simulink model "pokus05_serial_port"  (R2023a)
settings: Solver=VariableStepDiscrete  StartTime=0.0  StopTime=inf  RelTol=1e-3
undefined symbols (not defined in the file): UartDataRx, UartDataRx_Active
libraries: Miscellaneous x18, Memory_Blocks_Lib x7, Counters_Lib x4, Bit_Multiplexers_Lib x3, Decoders_Lib x2, Garbage x1, simulink_extras x1
settings Model: PacingRate=100  Creator=Jozko Mrkvicka  LastModifiedBy=Jozko Mrkvicka

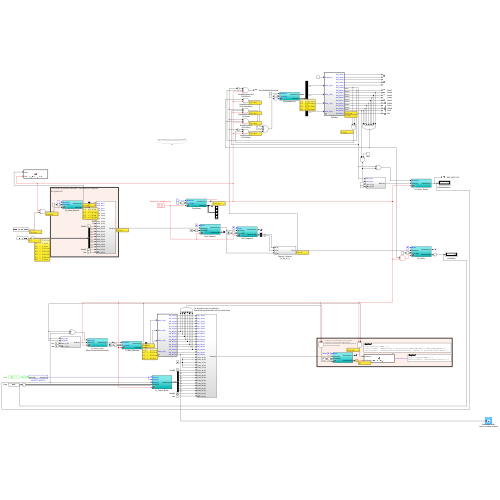
[thumbnail: Simulink's stored preview of the top-level diagram]
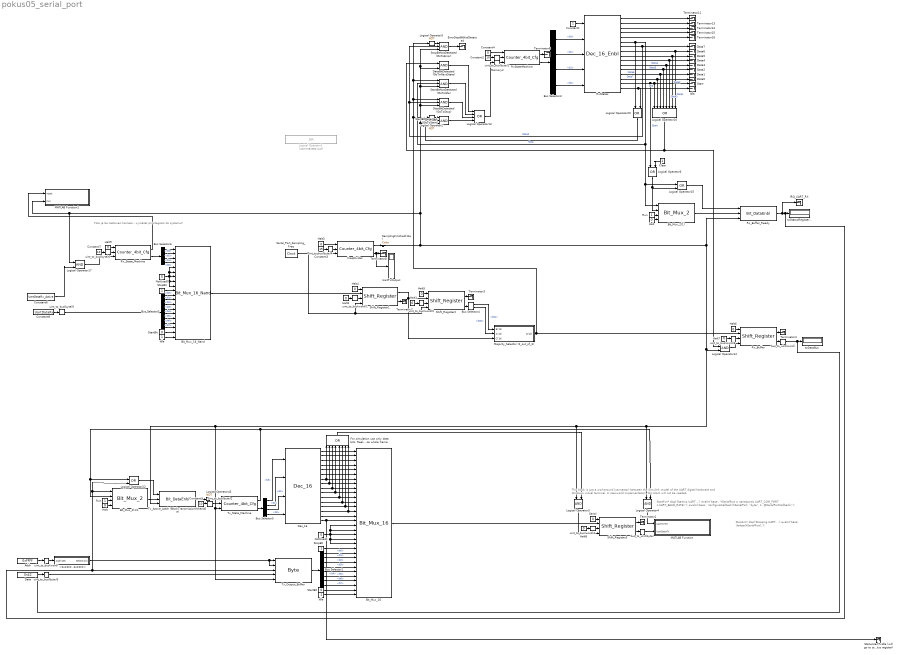
== system pokus05_serial_port ==
  note: Toto je len testovaci harness - vymazat pri integracii
      | do systemu!!
  note: StartFcn*
      | disp('Starting UART...')
      | evalin('base', 'hSerialPort = serialport(c.UART_COM_PORT, c.UART_BAUD_RATE);');
      | evalin('base', 'configureCallback(hSerialPort, "byte", 1, @SerialPortCallback);');
  note: StopFcn*
      | disp('Stopping UART...')
      | evalin('base', 'delete(hSerialPort);');
  note: This block is just a workaround (connector) between
      |                      the Simulink model of the UART digital hardware
      |                      and Windows virtual terminal. In real-world implementation,
      |                      this block will not be needed.
  "  Halt" : Constant  Value=0  OutDataTypeStr=boolean
  "  Idle" : Constant  OutDataTypeStr=boolean
   Halt{,3..6,9} (6 alike) : Constant  Value=0  OutDataTypeStr=boolean
   Halt{1..2,7..8} (4 alike) : Constant  Value=0  OutDataTypeStr=uint16
  " Idle" : Constant  OutDataTypeStr=boolean
  " Run" : Constant  OutDataTypeStr=boolean
  " StartBit" : Constant  Value=0  OutDataTypeStr=boolean
  " StopBit" : Constant  OutDataTypeStr=boolean
  <0xFFFF..0xFFFF> : Subsystem
  Addr : Constant  Value=0xFFFF  OutDataTypeStr=uint16
  Bit_Mux_16 : Bit_Multiplexers_Lib/Bit_Mux_16  SystemSampleTime=-1  VariantActivationTime=update diagram  Latency=0  AutoFrameSizeCalculation=off
  Bit_Mux_16_Nand : Garbage/Bit_Mux_16_Nand  SystemSampleTime=-1  VariantActivationTime=update diagram  Latency=0  AutoFrameSizeCalculation=off
  Bit_Mux_2(1) : Bit_Multiplexers_Lib/Bit_Mux_2  SystemSampleTime=-1  VariantActivationTime=update diagram  Latency=0  AutoFrameSizeCalculation=off
  Bit_Mux_2(1)1 : Bit_Multiplexers_Lib/Bit_Mux_2  SystemSampleTime=-1  VariantActivationTime=update diagram  Latency=0  AutoFrameSizeCalculation=off
  Bus Selector1 : BusSelector  OutputSignals=b0,b1,b2,b3,b4,b5,b6,b7
  Bus Selector2 : BusSelector  OutputSignals=b0,b1,b2,b3,b4,b5,b6,b7
  Bus Selector3 : BusSelector  OutputSignals=b3,b2,b1,b0
  Bus Selector4 : BusSelector  OutputSignals=b01,b00
  Bus Selector5 : BusSelector  OutputSignals=b3,b2,b1,b0
  Bus Selector6 : BusSelector  OutputSignals=b3,b2,b1,b0
  Clear : Constant  OutDataTypeStr=boolean
  Constant1 : Constant  OutDataTypeStr=boolean
  Constant2 : Constant  Value=10  OutDataTypeStr=uint8
  Constant3 : Constant  Value=15  OutDataTypeStr=uint8
  Constant4 : Constant  Value=0  OutDataTypeStr=boolean
  Constant5 : Constant  Value=10  OutDataTypeStr=uint8
  Constant6 : Constant  Value=UartDataRx_Active  OutDataTypeStr=boolean
  Constant7 : Constant  Value=10  OutDataTypeStr=uint8
  Constant8 : Constant  Value=UartDataRx  OutDataTypeStr=uint8
  Data : Constant  Value=0x42  OutDataTypeStr=uint8
  Data{0..7} (8 alike) : Terminator
  DataBitDetected (GoToNextState) : Logic  IconShape=distinctive  AllPortsSameDT=off  OutDataTypeStr=boolean
  Dec_16 : Decoders_Lib/Dec_16  SystemSampleTime=-1  VariantActivationTime=update diagram  Latency=0  AutoFrameSizeCalculation=off
  ErrorStopBitNotDetected : Terminator
  For simulation use only data bits. Real-world implementation will use whole frame. : Logic  Operator=OR  Inputs=8  IconShape=distinctive  AllPortsSameDT=off  OutDataTypeStr=boolean
  FreqDivider : Counters_Lib/Counter_4bit_Cfg  SystemSampleTime=-1  VariantActivationTime=update diagram  Latency=0  AutoFrameSizeCalculation=off
  IRQ_UART_RX : Terminator
  Idle : Terminator
  Logical Operator1 : Logic  Commented=on  Operator=OR  Inputs=16  IconShape=distinctive  OutDataTypeStr=boolean
  Logical Operator10 : Logic  Operator=OR  Inputs=8  IconShape=distinctive  AllPortsSameDT=off  OutDataTypeStr=boolean
  Logical Operator{3..4,12,17} (4 alike) : Logic  IconShape=distinctive  AllPortsSameDT=off  OutDataTypeStr=boolean
  Logical Operator13 : Logic  Operator=OR  Inputs=4  IconShape=distinctive  AllPortsSameDT=off  OutDataTypeStr=boolean
  Logical Operator{6,15,20,22} (4 alike) : Logic  Operator=OR  IconShape=distinctive  AllPortsSameDT=off  OutDataTypeStr=boolean
  Logical Operator2 : Logic  Operator=NOT  IconShape=distinctive  AllPortsSameDT=off  OutDataTypeStr=boolean
  Logical Operator43 : Logic  Operator=NOT  IconShape=distinctive  AllPortsSameDT=off  OutDataTypeStr=boolean
  Logical Operator5 : Logic  Operator=NOT  IconShape=distinctive  AllPortsSameDT=off  OutDataTypeStr=boolean
  MATLAB Function : MATLAB Function  StartFcn=|  StopFcn=|  TreatAsAtomicUnit=on  SystemSampleTime=1
      StartFcn=|
      | disp('Starting UART...')
      | evalin('base', 'hSerialPort = serialport(c.UART_COM_PORT, c.UART_BAUD_RATE);');
      | evalin('base', 'configureCallback(hSerialPort, "byte", 1, @SerialPortCallback);');
      StopFcn=|
      | disp('Stopping UART...')
      | evalin('base', 'delete(hSerialPort);');
  MATLAB Function1 : MATLAB Function  TreatAsAtomicUnit=on
  Majority_Selector (2_out_of_3) : Subsystem
  Memory2 : Memory
  NotUsed0 : Constant  Value=0  OutDataTypeStr=boolean
  NotUsed1 : Constant  Value=0  OutDataTypeStr=boolean
  Run : Constant  OutDataTypeStr=boolean
  RxStateMachine : Counters_Lib/Counter_4bit_Cfg  SystemSampleTime=-1  VariantActivationTime=update diagram  Latency=0  AutoFrameSizeCalculation=off
  RxStates : Decoders_Lib/Dec_16_Enbl  SystemSampleTime=-1  VariantActivationTime=update diagram  Latency=0  AutoFrameSizeCalculation=off
  Rx_Buffer : Memory_Blocks_Lib/Shift_Register  SystemSampleTime=-1  VariantActivationTime=update diagram  Latency=0  AutoFrameSizeCalculation=off
  Rx_Buffer_Ready : Memory_Blocks_Lib/Bit_DataEnbl  SystemSampleTime=-1  VariantActivationTime=update diagram  Latency=0  AutoFrameSizeCalculation=off
  "Rx_State_Machine " : Counters_Lib/Counter_4bit_Cfg  SystemSampleTime=-1  VariantActivationTime=update diagram  Latency=0  AutoFrameSizeCalculation=off
  SamplingFinished(16x) : Miscellaneous/Color  SystemSampleTime=-1  VariantActivationTime=update diagram  Latency=0  AutoFrameSizeCalculation=off
  Serial : Constant  Value=0  OutDataTypeStr=boolean
  Serial_Port_Sampling_Freq : simulink_extras/Flip Flops/Clock  period=1
  Shift_Register1 : Memory_Blocks_Lib/Shift_Register  SystemSampleTime=-1  VariantActivationTime=update diagram  Latency=0  AutoFrameSizeCalculation=off
  Shift_Register2 : Memory_Blocks_Lib/Shift_Register  SystemSampleTime=-1  VariantActivationTime=update diagram  Latency=0  AutoFrameSizeCalculation=off
  Shift_Register3 : Memory_Blocks_Lib/Shift_Register  SystemSampleTime=-1  VariantActivationTime=update diagram  Latency=0  AutoFrameSizeCalculation=off
  Start : Terminator
  StartBit : Constant  Value=0  OutDataTypeStr=boolean
  StartBitDetected (GoToStart) : Logic  Inputs=3  IconShape=distinctive  AllPortsSameDT=off  OutDataTypeStr=boolean
  StartBitNotDetected (GoToIdle) : Logic  Inputs=3  IconShape=distinctive  AllPortsSameDT=off  OutDataTypeStr=boolean
  StatusUartTxIdle (will go to status register) : Terminator
  StopBit : Constant  OutDataTypeStr=boolean
  StopBitDetected (GoToStop) : Logic  Inputs=3  IconShape=distinctive  AllPortsSameDT=off  OutDataTypeStr=boolean
  StopBitNotDetected (GoToError) : Logic  Inputs=3  IconShape=distinctive  AllPortsSameDT=off  OutDataTypeStr=boolean
  Terminator{1,3..4,6..8,11,13..16} (11 alike) : Terminator
  Tx_Active_Latch (BlockTransmissionWhenIdle) : Memory_Blocks_Lib/Bit_DataEnbl  SystemSampleTime=-1  VariantActivationTime=update diagram  Latency=0  AutoFrameSizeCalculation=off
  Tx_Output_Buffer : Memory_Blocks_Lib/Byte  SystemSampleTime=-1  VariantActivationTime=update diagram  Latency=0  AutoFrameSizeCalculation=off
  Tx_State_Machine : Counters_Lib/Counter_4bit_Cfg  SystemSampleTime=-1  VariantActivationTime=update diagram  Latency=0  AutoFrameSizeCalculation=off
  UartTxOutput : Display
  bus_to_uint(byte) : Miscellaneous/bus_to_uint(byte)
  bus_to_uint(word) : Miscellaneous/bus_to_uint(word)
  toDataBus : Display
  toStatusRegister... : Display
  uint_to_bus(byte){1..6} (6 alike) : Miscellaneous/uint_to_bus(byte)  SystemSampleTime=-1  VariantActivationTime=update diagram  Latency=0  AutoFrameSizeCalculation=off
  uint_to_bus(word){,1..4} (5 alike) : Miscellaneous/uint_to_bus(word)
  wires:
  SamplingFinished(16x)/1 -> Logical Operator4/1, Tx_Active_Latch (BlockTransmissionWhenIdle)/3, Tx_State_Machine/3, Tx_Output_Buffer/5, Logical Operator3/1, Logical Operator12/2, Rx_Buffer_Ready/3, MATLAB Function1/2(CLK), Logical Operator17/1, StopBitNotDetected (GoToError)/3, DataBitDetected (GoToNextState)/2, StartBitNotDetected (GoToIdle)/3, StopBitDetected (GoToStop)/3, StartBitDetected (GoToStart)/3
  Shift_Register1/2 -> Terminator7/1
  Shift_Register2/1 -> Terminator3/1
  Bus Selector4/2 -> Majority_Selector (2_out_of_3)/2(A(1b))  "<b00>"
  Bus Selector4/1 -> Majority_Selector (2_out_of_3)/1(B(1b))  "<b01>"
  Majority_Selector (2_out_of_3)/1(D(1b)) -> Rx_Buffer/2, Logical Operator2/1, Logical Operator5/1, StartBitNotDetected (GoToIdle)/1, StopBitDetected (GoToStop)/1
  Rx_Buffer/2 -> bus_to_uint(word)/1
  RxStates/16 -> Idle/1, Logical Operator20/2  "Idle"
  RxStates/15 -> Logical Operator6/1, Logical Operator10/1, Start/1  "Start"
  RxStates/14 -> Logical Operator10/2, Data0/1  "Data7"
  RxStates/13 -> Logical Operator10/3, Data1/1  "Data6"
  RxStates/12 -> Logical Operator10/4, Data2/1  "Data5"
  RxStates/11 -> Logical Operator10/5, Data3/1  "Data4"
  RxStates/10 -> Logical Operator10/6, Data4/1  "Data3"
  RxStates/9 -> Logical Operator10/7, Data5/1  "Data2"
  RxStates/8 -> Logical Operator10/8, Data6/1  "Data1"
  RxStates/7 -> StopBitDetected (GoToStop)/2, StopBitNotDetected (GoToError)/2, Data7/1  "Data0"
  RxStates/6 -> Logical Operator20/1, Logical Operator15/1, Bit_Mux_2(1)/1, StartBitNotDetected (GoToIdle)/2  "Stop"
  RxStates/1 -> Terminator11/1
  RxStates/2 -> Terminator13/1
  RxStates/3 -> Terminator14/1
  RxStates/5 -> Terminator16/1
  RxStates/4 -> Terminator15/1
  RxStateMachine/2 -> Bus Selector3/1
  Bus Selector3/1 -> RxStates/2  "<b3>"
  Bus Selector3/2 -> RxStates/3  "<b2>"
  Bus Selector3/3 -> RxStates/4  "<b1>"
  Bus Selector3/4 -> RxStates/5  "<b0>"
  Logical Operator2/1 -> StartBitDetected (GoToStart)/1
  Logical Operator13/1 -> Memory2/1
  StartBitDetected (GoToStart)/1 -> Logical Operator13/4
  StopBitDetected (GoToStop)/1 -> Logical Operator13/3
  Logical Operator5/1 -> StopBitNotDetected (GoToError)/1
  StopBitNotDetected (GoToError)/1 -> ErrorStopBitNotDetected/1
  StartBitNotDetected (GoToIdle)/1 -> Logical Operator13/2
  DataBitDetected (GoToNextState)/1 -> Logical Operator13/1
  Logical Operator12/1 -> Rx_Buffer/4
  Constant2/1 -> uint_to_bus(byte)1/1
  uint_to_bus(byte)1/1 -> RxStateMachine/2
  RxStateMachine/1 -> Terminator6/1
  Constant4/1 -> RxStateMachine/1
  Constant8/1 -> uint_to_bus(byte)5/1
  Logical Operator20/1 -> StartBitDetected (GoToStart)/2
  Logical Operator10/1 -> DataBitDetected (GoToNextState)/1, Logical Operator12/1
  Memory2/1 -> RxStateMachine/3
  NotUsed0/1 -> Bit_Mux_16_Nand/5, Bit_Mux_16_Nand/6, Bit_Mux_16_Nand/7, Bit_Mux_16_Nand/8, Bit_Mux_16_Nand/9
  Bit_Mux_16_Nand/1 -> Shift_Register1/2
  Constant1/1 -> RxStates/1
  Addr/1 -> uint_to_bus(word)/1
  uint_to_bus(word)/1 -> <0xFFFF..0xFFFF>/1(Addr(2B))
  Shift_Register1/1 -> Shift_Register2/2, Majority_Selector (2_out_of_3)/3(C(1b))
  " Run"/1 -> Bit_Mux_2(1)/3
  " Halt"/1 -> Bit_Mux_2(1)/4
  Bit_Mux_2(1)/1 -> Rx_Buffer_Ready/2
  Rx_Buffer_Ready/1 -> toStatusRegister.../1, Bit_Mux_2(1)1/1, Logical Operator22/2, Tx_Output_Buffer/3, IRQ_UART_RX/1
  Logical Operator15/1 -> Rx_Buffer_Ready/1
  " Halt2"/1 -> uint_to_bus(word)1/1
  uint_to_bus(word)3/1 -> Rx_Buffer/3
  " Halt4"/1 -> Shift_Register1/1
  " Halt5"/1 -> Shift_Register2/1
  " Halt6"/1 -> Rx_Buffer/1
  Shift_Register2/2 -> Bus Selector4/1
  uint_to_bus(word)1/1 -> Shift_Register1/3
  " Halt1"/1 -> uint_to_bus(word)2/1
  uint_to_bus(word)2/1 -> Shift_Register2/3
  " Halt7"/1 -> uint_to_bus(word)3/1
  Rx_Buffer/1 -> Terminator4/1
  bus_to_uint(word)/1 -> uint_to_bus(byte)3/1, toDataBus/1
  Bit_Mux_16/1 -> Shift_Register3/2
  Serial_Port_Sampling_Freq/1 -> Shift_Register2/4, Shift_Register1/4, FreqDivider/3
  <0xFFFF..0xFFFF>/1(Select(1b)) -> Tx_Output_Buffer/1, Tx_Output_Buffer/2
  Tx_Output_Buffer/1 -> Bus Selector1/1
  Tx_State_Machine/2 -> Bus Selector5/1
  Logical Operator43/1 -> Tx_State_Machine/1
  Tx_State_Machine/1 -> Logical Operator4/2, Bit_Mux_2(1)1/2, Logical Operator22/1
  uint_to_bus(byte)2/1 -> Tx_State_Machine/2
  Constant5/1 -> uint_to_bus(byte)2/1
  Bus Selector5/1 -> Dec_16/1  "<b3>"
  Bus Selector5/2 -> Dec_16/2  "<b2>"
  Bus Selector5/3 -> Dec_16/3  "<b1>"
  Bus Selector5/4 -> Dec_16/4  "<b0>"
  "  Halt"/1 -> Bit_Mux_2(1)1/4
  Run/1 -> Bit_Mux_2(1)1/3
  Logical Operator22/1 -> Tx_Active_Latch (BlockTransmissionWhenIdle)/1
  Bit_Mux_2(1)1/1 -> Tx_Active_Latch (BlockTransmissionWhenIdle)/2
  Tx_Active_Latch (BlockTransmissionWhenIdle)/1 -> Logical Operator43/1
  FreqDivider/1 -> SamplingFinished(16x)/1
  Dec_16/1 -> Bit_Mux_16/1
  Dec_16/2 -> Bit_Mux_16/2
  Dec_16/3 -> Bit_Mux_16/3
  Dec_16/4 -> Bit_Mux_16/4
  Dec_16/5 -> Bit_Mux_16/5
  Dec_16/6 -> Bit_Mux_16/6
  Dec_16/7 -> Bit_Mux_16/7, For simulation use only data bits. Real-world implementation will use whole frame./1
  Dec_16/8 -> For simulation use only data bits. Real-world implementation will use whole frame./2, Bit_Mux_16/8
  Dec_16/9 -> Bit_Mux_16/9, For simulation use only data bits. Real-world implementation will use whole frame./3
  Dec_16/10 -> For simulation use only data bits. Real-world implementation will use whole frame./4, Bit_Mux_16/10
  Dec_16/11 -> For simulation use only data bits. Real-world implementation will use whole frame./5, Bit_Mux_16/11
  Dec_16/12 -> For simulation use only data bits. Real-world implementation will use whole frame./6, Bit_Mux_16/12
  Dec_16/13 -> For simulation use only data bits. Real-world implementation will use whole frame./7, Bit_Mux_16/13
  Dec_16/14 -> For simulation use only data bits. Real-world implementation will use whole frame./8, Bit_Mux_16/14
  Dec_16/15 -> Bit_Mux_16/15
  Dec_16/16 -> StatusUartTxIdle (will go to status register)/1, Bit_Mux_16/16
  FreqDivider/2 -> UartTxOutput/1, Terminator8/1
  Constant3/1 -> uint_to_bus(byte)4/1
  uint_to_bus(byte)4/1 -> FreqDivider/2
  " Halt3"/1 -> FreqDivider/1
  " Halt8"/1 -> uint_to_bus(word)4/1
  uint_to_bus(word)4/1 -> Shift_Register3/3
  Shift_Register3/1 -> Terminator1/1
  Serial/1 -> Shift_Register3/1
  Shift_Register3/2 -> bus_to_uint(byte)/1
  bus_to_uint(byte)/1 -> MATLAB Function/2(UartDataTx)
  For simulation use only data bits. Real-world implementation will use whole frame./1 -> Logical Operator3/2
  Logical Operator3/1 -> Shift_Register3/4
  NotUsed1/1 -> Bit_Mux_16/19, Bit_Mux_16/21, Bit_Mux_16/20, Bit_Mux_16/17, Bit_Mux_16/18
  " StopBit"/1 -> Bit_Mux_16/22
  " Idle"/1 -> Bit_Mux_16/32
  " StartBit"/1 -> Bit_Mux_16/31
  Bus Selector1/8 -> Bit_Mux_16/30  "<b7>"
  Bus Selector1/7 -> Bit_Mux_16/29  "<b6>"
  Bus Selector1/6 -> Bit_Mux_16/28  "<b5>"
  Bus Selector1/5 -> Bit_Mux_16/27  "<b4>"
  Bus Selector1/4 -> Bit_Mux_16/26  "<b3>"
  Bus Selector1/3 -> Bit_Mux_16/25  "<b2>"
  Bus Selector1/2 -> Bit_Mux_16/24  "<b1>"
  Bus Selector1/1 -> Bit_Mux_16/23  "<b0>"
  uint_to_bus(byte)3/1 -> Tx_Output_Buffer/4
  Logical Operator4/1 -> MATLAB Function/1(UartWrite)
  StartBit/1 -> Bit_Mux_16_Nand/19
  Bus Selector2/7 -> Bit_Mux_16_Nand/17  "<b6>"
  Bus Selector2/3 -> Bit_Mux_16_Nand/13  "<b2>"
  StopBit/1 -> Bit_Mux_16_Nand/10
  Bus Selector2/5 -> Bit_Mux_16_Nand/15  "<b4>"
  Bus Selector2/4 -> Bit_Mux_16_Nand/14  "<b3>"
  Bus Selector2/2 -> Bit_Mux_16_Nand/12  "<b1>"
  Bus Selector2/6 -> Bit_Mux_16_Nand/16  "<b5>"
  Bus Selector2/1 -> Bit_Mux_16_Nand/11  "<b0>"
  uint_to_bus(byte)5/1 -> Bus Selector2/1
  Bus Selector2/8 -> Bit_Mux_16_Nand/18  "<b7>"
  "  Idle"/1 -> Bit_Mux_16_Nand/20
  "Rx_State_Machine "/2 -> Bus Selector6/1
  Bus Selector6/1 -> Bit_Mux_16_Nand/1  "<b3>"
  Bus Selector6/2 -> Bit_Mux_16_Nand/2  "<b2>"
  Bus Selector6/3 -> Bit_Mux_16_Nand/3  "<b1>"
  Bus Selector6/4 -> Bit_Mux_16_Nand/4  "<b0>"
  " Halt9"/1 -> "Rx_State_Machine "/1
  uint_to_bus(byte)6/1 -> "Rx_State_Machine "/2
  Constant7/1 -> uint_to_bus(byte)6/1
  Logical Operator17/1 -> "Rx_State_Machine "/3
  Constant6/1 -> Logical Operator17/2
  "Rx_State_Machine "/1 -> MATLAB Function1/1(reset)
  Logical Operator6/1 -> Logical Operator15/2, Bit_Mux_2(1)/2
  Clear/1 -> Logical Operator6/2

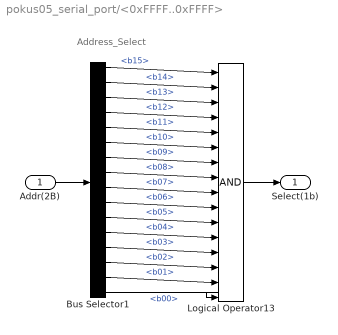
== system pokus05_serial_port/<0xFFFF..0xFFFF> ==
  note: Address_Select
  Addr(2B) : Inport
  Bus Selector1 : BusSelector  OutputSignals=b15,b14,b13,b12,b11,b10,b09,b08,b07,b06,b05,b04,b03,b02,b01,b00
  Logical Operator13 : Logic  Inputs=16  IconShape=distinctive  AllPortsSameDT=off  OutDataTypeStr=boolean
  Select(1b) : Outport
  wires:
  Logical Operator13/1 -> Select(1b)/1
  Addr(2B)/1 -> Bus Selector1/1
  Bus Selector1/15 -> Logical Operator13/15  "<b01>"
  Bus Selector1/7 -> Logical Operator13/7  "<b09>"
  Bus Selector1/13 -> Logical Operator13/13  "<b03>"
  Bus Selector1/11 -> Logical Operator13/11  "<b05>"
  Bus Selector1/9 -> Logical Operator13/9  "<b07>"
  Bus Selector1/6 -> Logical Operator13/6  "<b10>"
  Bus Selector1/8 -> Logical Operator13/8  "<b08>"
  Bus Selector1/3 -> Logical Operator13/3  "<b13>"
  Bus Selector1/10 -> Logical Operator13/10  "<b06>"
  Bus Selector1/4 -> Logical Operator13/4  "<b12>"
  Bus Selector1/14 -> Logical Operator13/14  "<b02>"
  Bus Selector1/12 -> Logical Operator13/12  "<b04>"
  Bus Selector1/16 -> Logical Operator13/16  "<b00>"
  Bus Selector1/5 -> Logical Operator13/5  "<b11>"
  Bus Selector1/1 -> Logical Operator13/1  "<b15>"
  Bus Selector1/2 -> Logical Operator13/2  "<b14>"

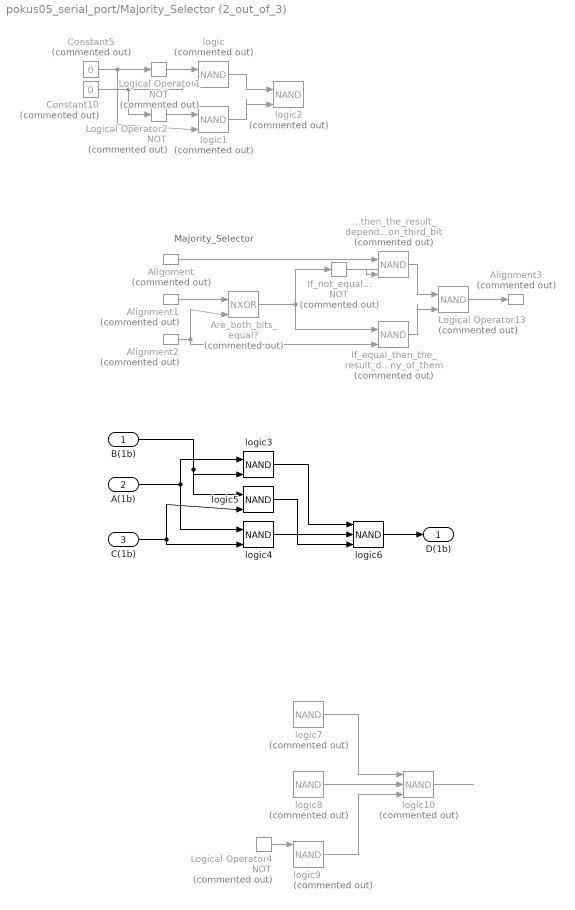
== system pokus05_serial_port/Majority_Selector (2_out_of_3) ==
  note: Majority_Selector
  B(1b) : Inport
  A(1b) : Inport  Port=2
  C(1b) : Inport  Port=3
  ...then_the_result_depends_only_on_third_bit : Logic  Commented=on  Operator=NAND  IconShape=distinctive  AllPortsSameDT=off  OutDataTypeStr=boolean
  Alignment{,1..3} (4 alike) : Miscellaneous/Alignment  Commented=on  SystemSampleTime=-1  VariantActivationTime=update diagram  Latency=0  AutoFrameSizeCalculation=off
  Are_both_bits_equal? : Logic  Commented=on  Operator=NXOR  IconShape=distinctive  AllPortsSameDT=off  OutDataTypeStr=boolean
  Constant10 : Constant  Commented=on  Value=0  OutDataTypeStr=boolean
  Constant5 : Constant  Commented=on  Value=0  OutDataTypeStr=boolean
  If_equal_then_the_result_depends_on_any_of_them : Logic  Commented=on  Operator=NAND  IconShape=distinctive  AllPortsSameDT=off  OutDataTypeStr=boolean
  If_not_equal... : Logic  Commented=on  Operator=NOT  IconShape=distinctive  AllPortsSameDT=off  OutDataTypeStr=boolean
  Logical Operator1 : Logic  Commented=on  Operator=NOT  IconShape=distinctive  AllPortsSameDT=off  OutDataTypeStr=boolean
  Logical Operator13 : Logic  Commented=on  Operator=NAND  IconShape=distinctive  AllPortsSameDT=off  OutDataTypeStr=boolean
  Logical Operator2 : Logic  Commented=on  Operator=NOT  IconShape=distinctive  AllPortsSameDT=off  OutDataTypeStr=boolean
  Logical Operator4 : Logic  Commented=on  Operator=NOT  IconShape=distinctive  AllPortsSameDT=off  OutDataTypeStr=boolean
  logic{,1..2,7..8} (5 alike) : Logic  Commented=on  Operator=NAND  IconShape=distinctive  AllPortsSameDT=off  OutDataTypeStr=boolean
  logic10 : Logic  Commented=on  Operator=NAND  Inputs=3  IconShape=distinctive  AllPortsSameDT=off  OutDataTypeStr=boolean
  logic3 : Logic  Operator=NAND  IconShape=distinctive  AllPortsSameDT=off  OutDataTypeStr=boolean
  logic4 : Logic  Operator=NAND  IconShape=distinctive  AllPortsSameDT=off  OutDataTypeStr=boolean
  logic5 : Logic  Operator=NAND  IconShape=distinctive  AllPortsSameDT=off  OutDataTypeStr=boolean
  logic6 : Logic  Operator=NAND  Inputs=3  IconShape=distinctive  AllPortsSameDT=off  OutDataTypeStr=boolean
  logic9 : Logic  Commented=on  Operator=NAND  Inputs=3  IconShape=distinctive  AllPortsSameDT=off  OutDataTypeStr=boolean
  D(1b) : Outport
  wires:
  Logical Operator13/1 -> Alignment3/1
  If_equal_then_the_result_depends_on_any_of_them/1 -> Logical Operator13/2
  Are_both_bits_equal?/1 -> If_not_equal.../1, If_equal_then_the_result_depends_on_any_of_them/1
  If_not_equal.../1 -> ...then_the_result_depends_only_on_third_bit/2
  ...then_the_result_depends_only_on_third_bit/1 -> Logical Operator13/1
  Alignment/1 -> ...then_the_result_depends_only_on_third_bit/1
  Alignment1/1 -> Are_both_bits_equal?/1
  Alignment2/1 -> Are_both_bits_equal?/2, If_equal_then_the_result_depends_on_any_of_them/2
  logic6/1 -> D(1b)/1
  Logical Operator1/1 -> logic/1
  Constant5/1 -> logic1/2, Logical Operator1/1
  Logical Operator2/1 -> logic1/1
  Constant10/1 -> Logical Operator2/1, logic/2
  logic/1 -> logic2/1
  logic1/1 -> logic2/2
  A(1b)/1 -> logic3/1, logic4/1
  B(1b)/1 -> logic5/1, logic3/2
  C(1b)/1 -> logic5/2, logic4/2
  logic4/1 -> logic6/2
  logic3/1 -> logic6/1
  logic5/1 -> logic6/3
  logic9/1 -> logic10/3
  logic10/1 -> ?
  logic7/1 -> logic10/1
  ? -> logic7/1, Logical Operator4/1, logic8/1
  Logical Operator4/1 -> logic9/1
  ? -> logic9/3, logic8/2
  ? -> logic7/2, logic9/2
  logic8/1 -> logic10/2

== matlab function pokus05_serial_port/MATLAB Function1 ==
  data: reset input boolean; CLK input
% function active = Rx_Active_Latch(set, reset)
%     persistent state;
%     if isempty(state)
%         state = false;
%     end
% 
%     coder.extrinsic('evalin');
%     coder.extrinsic('assignin');
% 
%     if (true == set) && (false == reset)
%         state = true;
%     end
% 
%     if (true == reset)
%         state = false;
%         evalin('base', 'Rx_Active_Latch = false');
%         % assignin('base', 'Rx_Active_Latch', Rx_Active_Latch);
%     end
% end

function Rx_Active_Latch(reset, CLK)
    persistent prevCLK;
    if isempty(prevCLK)
        prevCLK = false;
    end

    coder.extrinsic('evalin');
    coder.extrinsic('set_param');
    coder.extrinsic('gcs');
    % 
    % if (true == in)
    %     state = true;
    % end
    % 
    if (true == reset) && (true == prevCLK) && (false == CLK)
        evalin('base', 'UartDataRx_Active = false');
        set_param(gcs, 'SimulationCommand', 'update');
        % assignin('base', 'Rx_Active_Latch', Rx_Active_Latch);
    end

    prevCLK = CLK;
end

== matlab function pokus05_serial_port/MATLAB Function ==
  data: UartWrite input boolean; UartDataTx input uint8
function UartSendByte(UartWrite, UartDataTx)
    coder.extrinsic('evalin');
    coder.extrinsic('assignin');
    assignin('base', 'UartDataTx', UartDataTx);

    if (true == UartWrite)
        evalin('base', 'write(hSerialPort, UartDataTx, "uint8");');
    end
end
